simulink model "TorqueVect_HIL_CAN"  (R2022a)
settings: Solver=VariableStepAuto  StartTime=0.0  StopTime=300  RelTol=1e-3
PreLoadFcn:
  | run('Parameters\FSE_Parameters.m')
values from neighbouring files (symbols this model uses):
  Kd = 0;')    [open_carmaker_gui.m]
  Ki = 0    [open_carmaker_gui.m]
undefined symbols (not defined in the file or in its folder): BRegenEnabledButton, canChannel, CyalphaLookUp, efficiency, Fz_curve, Fz_scaling_long, gearR, izz, jw, kd, ki, Kp, kp, l_f, l_r, lambda, m, Mz_max, N, N_lat, N_long, P_max, pid_kd_lat, pid_kd_long, pid_ki_lat, pid_ki_long, pid_kp_lat, pid_kp_long, R_max, rw, steerR, T_i_max, TC_Decr_Gas, TC_Derivative, TC_Incr_Gas, TC_On, TC_Relay_Off, TC_Relay_On, tireCornerStiffness, Ts, TV_On, TV_Override, velocity_lookup, velocity_lookup_lat, y_ref, yrr_scaling
libraries: simulink x218, slpidlib x135, CarMaker4SL x73, TractionControlLibrary x13, canmsglib x11, canlib x10, TorqueVectoringLibrary x6, simulink_extras x4, PedalConversionLibrary x3, PowerControlLibrary x1
(part 2 of 26)

== system TorqueVect_HIL_CAN/CarMaker/IPG Vehicle/CarAndTrailer/Forces/Tires ==
  note: The TireXX_Out signals will only be used if FileIdent is "CarMaker-Tire-CM4SL" in the tire parameter file!
      | An example parameter file can be found in Data/Tire/DT_CM4SL_UserTire.
  Sync_In : Inport
  TireFL_In : Inport  Port=2
  TireFR_In : Inport  Port=3
  TireRL_In : Inport  Port=4
  TireRR_In : Inport  Port=5
  Bus Creator{1..4} (4 alike) : BusCreator  Inputs=11
  Demux{1..3,8} (4 alike) : Demux  Outputs=7
      settings: DisplayOption=none
  TireFL : Subsystem
  TireFR : Subsystem
  TireRL : Subsystem
  TireRR : Subsystem
  TireFL_Out : Outport
  TireFR_Out : Outport  Port=2
  TireRL_Out : Outport  Port=3
  TireRR_Out : Outport  Port=4
  tag scope: TireFL=global, TireFR=global, TireRL=global, TireRR=global
  wires:
  Sync_In/1 -> TireRR/1(Sync_In), TireRL/1(Sync_In), TireFR/1(Sync_In), TireFL/1(Sync_In)
  Bus Creator4/1 -> TireRR_Out/1
  Bus Creator2/1 -> TireRL_Out/1
  Bus Creator1/1 -> TireFR_Out/1
  Demux3/5 -> TireRR/6(Rim_turnv)  "Tire_In Rim_turnv"
  Demux3/4 -> TireRR/5(Rim_rotv)  "Tire_In Rim_rotv"
  Demux3/1 -> [TireRR], TireRR/2(Load)  "Tire_In Load"
  Demux3/7 -> TireRR/8(muRoad)  "Tire_In mu"
  Demux3/6 -> TireRR/7(InclinAngle)  "Tire_In Camber"
  Demux3/2 -> TireRR/3(vxtrans)  "Tire_In vxtrans"
  Demux3/3 -> TireRR/4(vytrans)  "Tire_In vytrans"
  TireRR/11(AlignTrq) -> Bus Creator4/11  "Tire_Out AlignTrq"
  TireRR/10(RollResist) -> Bus Creator4/10  "Tire_Out RollResist"
  TireRR/9(OverturnTrq) -> Bus Creator4/9  "Tire_Out OverturnTrq"
  TireRR/8(LoadFrc) -> Bus Creator4/8  "Tire_Out LoadFrc"
  TireRR/7(SideFrc) -> Bus Creator4/7  "Tire_Out SideFrc"
  TireRR/6(LongFrc) -> Bus Creator4/6  "Tire_Out LongFrc"
  TireRR/5(vBelt) -> Bus Creator4/5  "Tire_Out vBelt"
  TireRR/4(rBelt_eff) -> Bus Creator4/4  "Tire_Out rBelt_eff"
  TireRR/3(TurnSlp) -> Bus Creator4/3  "Tire_Out TurnSlp"
  TireRR/1(Slp) -> Bus Creator4/1  "Tire_Out Slp"
  TireRR/2(Alpha) -> Bus Creator4/2  "Tire_Out Alpha"
  Demux2/5 -> TireRL/6(Rim_turnv)  "Tire_In Rim_turnv"
  Demux2/4 -> TireRL/5(Rim_rotv)  "Tire_In Rim_rotv"
  Demux2/1 -> [TireRL], TireRL/2(Load)  "Tire_In Load"
  Demux2/7 -> TireRL/8(muRoad)  "Tire_In mu"
  Demux2/6 -> TireRL/7(InclinAngle)  "Tire_In Camber"
  Demux2/2 -> TireRL/3(vxtrans)  "Tire_In vxtrans"
  Demux2/3 -> TireRL/4(vytrans)  "Tire_In vytrans"
  TireRL/11(AlignTrq) -> Bus Creator2/11  "Tire_Out AlignTrq"
  TireRL/10(RollResist) -> Bus Creator2/10  "Tire_Out RollResist"
  TireRL/9(OverturnTrq) -> Bus Creator2/9  "Tire_Out OverturnTrq"
  TireRL/8(LoadFrc) -> Bus Creator2/8  "Tire_Out LoadFrc"
  TireRL/7(SideFrc) -> Bus Creator2/7  "Tire_Out SideFrc"
  TireRL/6(LongFrc) -> Bus Creator2/6  "Tire_Out LongFrc"
  TireRL/5(vBelt) -> Bus Creator2/5  "Tire_Out vBelt"
  TireRL/4(rBelt_eff) -> Bus Creator2/4  "Tire_Out rBelt_eff"
  TireRL/3(TurnSlp) -> Bus Creator2/3  "Tire_Out TurnSlp"
  TireRL/1(Slp) -> Bus Creator2/1  "Tire_Out Slp"
  TireRL/2(Alpha) -> Bus Creator2/2  "Tire_Out Alpha"
  Demux1/5 -> TireFR/6(Rim_turnv)  "Tire_In Rim_turnv"
  Demux1/4 -> TireFR/5(Rim_rotv)  "Tire_In Rim_rotv"
  Demux1/1 -> [TireFR], TireFR/2(Load)  "Tire_In Load"
  Demux1/7 -> TireFR/8(muRoad)  "Tire_In mu"
  Demux1/6 -> TireFR/7(InclinAngle)  "Tire_In Camber"
  Demux1/2 -> TireFR/3(vxtrans)  "Tire_In vxtrans"
  Demux1/3 -> TireFR/4(vytrans)  "Tire_In vytrans"
  TireFR/11(AlignTrq) -> Bus Creator1/11  "Tire_Out AlignTrq"
  TireFR/10(RollResist) -> Bus Creator1/10  "Tire_Out RollResist"
  TireFR/9(OverturnTrq) -> Bus Creator1/9  "Tire_Out OverturnTrq"
  TireFR/8(LoadFrc) -> Bus Creator1/8  "Tire_Out LoadFrc"
  TireFR/7(SideFrc) -> Bus Creator1/7  "Tire_Out SideFrc"
  TireFR/6(LongFrc) -> Bus Creator1/6  "Tire_Out LongFrc"
  TireFR/5(vBelt) -> Bus Creator1/5  "Tire_Out vBelt"
  TireFR/4(rBelt_eff) -> Bus Creator1/4  "Tire_Out rBelt_eff"
  TireFR/3(TurnSlp) -> Bus Creator1/3  "Tire_Out TurnSlp"
  TireFR/1(Slp) -> Bus Creator1/1  "Tire_Out Slp"
  TireFR/2(Alpha) -> Bus Creator1/2  "Tire_Out Alpha"
  Demux8/5 -> TireFL/6(Rim_turnv)  "Tire_In Rim_turnv"
  Demux8/4 -> TireFL/5(Rim_rotv)  "Tire_In Rim_rotv"
  TireFL_In/1 -> Demux8/1
  Demux8/1 -> [TireFL], TireFL/2(Load)  "Tire_In Load"
  Demux8/7 -> TireFL/8(muRoad)  "Tire_In mu"
  Demux8/6 -> TireFL/7(InclinAngle)  "Tire_In Camber"
  Demux8/2 -> TireFL/3(vxtrans)  "Tire_In vxtrans"
  Demux8/3 -> TireFL/4(vytrans)  "Tire_In vytrans"
  TireFL/11(AlignTrq) -> Bus Creator3/11  "Tire_Out AlignTrq"
  TireFL/10(RollResist) -> Bus Creator3/10  "Tire_Out RollResist"
  TireFL/9(OverturnTrq) -> Bus Creator3/9  "Tire_Out OverturnTrq"
  TireFL/8(LoadFrc) -> Bus Creator3/8  "Tire_Out LoadFrc"
  TireFL/7(SideFrc) -> Bus Creator3/7  "Tire_Out SideFrc"
  TireFL/6(LongFrc) -> Bus Creator3/6  "Tire_Out LongFrc"
  TireFL/5(vBelt) -> Bus Creator3/5  "Tire_Out vBelt"
  TireFL/4(rBelt_eff) -> Bus Creator3/4  "Tire_Out rBelt_eff"
  TireFL/3(TurnSlp) -> Bus Creator3/3  "Tire_Out TurnSlp"
  TireFL/1(Slp) -> Bus Creator3/1  "Tire_Out Slp"
  TireFL/2(Alpha) -> Bus Creator3/2  "Tire_Out Alpha"
  Bus Creator3/1 -> TireFL_Out/1
  TireFR_In/1 -> Demux1/1
  TireRL_In/1 -> Demux2/1
  TireRR_In/1 -> Demux3/1

== system TorqueVect_HIL_CAN/CarMaker/IPG Vehicle/CarAndTrailer/Forces/Vehicle Forces ==
  Sync_In : Inport
  Bus Creator1 : BusCreator  Inputs=12
  Bus Creator8 : BusCreator  Inputs=16
  BusCreator1 : BusCreator  Inputs=4
  BusCreator2 : BusCreator  Inputs=9
  Demux : Demux  Outputs=16
      settings: DisplayOption=none
  Demux1 : Demux  Outputs=12
      settings: DisplayOption=none
  Demux2 : Demux  Outputs=13
      settings: DisplayOption=none
  Forces : S-Function  FunctionName=CM_Sfun  Parameters='Forces'  SFunctionDeploymentMode=off  EnableBusSupport=off
  Terminator : Terminator
  Sync_Out : Outport
  Car.Virtual : Outport  Port=2
  Car.Aero : Outport  Port=3
  Car.Load : Outport  Port=4
  wires:
  BusCreator1/1 -> Terminator/1  "Aero IF (in)"
  Demux2/13 -> BusCreator2/9  "car Aero Trq_1 z"
  Demux2/12 -> BusCreator2/8  "car Aero Trq_1 y"
  Demux2/11 -> BusCreator2/7  "car Aero Trq_1 x"
  Demux2/10 -> BusCreator2/6  "car Aero Frc_1 z"
  Demux2/9 -> BusCreator2/5  "car Aero Frc_1 y"
  Demux2/8 -> BusCreator2/4  "car Aero Frc_1 x"
  Demux2/7 -> BusCreator2/3  "car Aero PoA_1 z"
  Demux2/6 -> BusCreator2/2  "car Aero PoA_1 y"
  Demux2/5 -> BusCreator2/1  "car Aero PoA_1 x"
  Demux2/4 -> BusCreator1/4  "car Aero tau_1"
  Demux2/3 -> BusCreator1/3  "car Aero ApproachVel_1 z"
  Demux2/2 -> BusCreator1/2  "car Aero ApproachVel_1 y"
  Demux2/1 -> BusCreator1/1  "car Aero ApproachVel_1 x"
  Demux/16 -> Bus Creator8/16  "Car Load_3 tz"
  Demux/15 -> Bus Creator8/15  "Car Load_3 ty"
  Demux/14 -> Bus Creator8/14  "Car Load_3 tx"
  Demux/13 -> Bus Creator8/13  "Car Load_3 mass"
  Demux1/12 -> Bus Creator1/12  "Car Virtual Trq_0 z"
  Demux1/11 -> Bus Creator1/11  "Car Virtual Trq_0 y"
  Demux1/10 -> Bus Creator1/10  "Car Virtual Trq_0 x"
  Demux1/9 -> Bus Creator1/9  "Car Virtual Trq_1 z"
  Demux1/8 -> Bus Creator1/8  "Car Virtual Trq_1 y"
  Demux1/7 -> Bus Creator1/7  "Car Virtual Trq_1 x"
  Demux1/6 -> Bus Creator1/6  "Car Virtual Frc_0 z"
  Demux1/5 -> Bus Creator1/5  "Car Virtual Frc_0 y"
  Demux1/4 -> Bus Creator1/4  "Car Virtual Frc_0 x"
  Sync_In/1 -> Forces/1
  Forces/1 -> Sync_Out/1
  BusCreator2/1 -> Car.Aero/1
  Demux1/1 -> Bus Creator1/1  "Car Virtual Frc_1 x"
  Demux1/2 -> Bus Creator1/2  "Car Virtual Frc_1 y"
  Demux1/3 -> Bus Creator1/3  "Car Virtual Frc_1 z"
  Forces/3 -> Demux2/1
  Forces/2 -> Demux1/1
  Bus Creator1/1 -> Car.Virtual/1
  Bus Creator8/1 -> Car.Load/1
  Demux/1 -> Bus Creator8/1  "Car Load_0 mass"
  Demux/2 -> Bus Creator8/2  "Car Load_0 tx"
  Demux/3 -> Bus Creator8/3  "Car Load_0 ty"
  Demux/4 -> Bus Creator8/4  "Car Load_0 tz"
  Demux/5 -> Bus Creator8/5  "Car Load_1 mass"
  Demux/6 -> Bus Creator8/6  "Car Load_1 tx"
  Demux/7 -> Bus Creator8/7  "Car Load_1 ty"
  Demux/8 -> Bus Creator8/8  "Car Load_1 tz"
  Demux/9 -> Bus Creator8/9  "Car Load_2 mass"
  Demux/10 -> Bus Creator8/10  "Car Load_2 tx"
  Demux/11 -> Bus Creator8/11  "Car Load_2 ty"
  Demux/12 -> Bus Creator8/12  "Car Load_2 tz"
  Forces/4 -> Demux/1

== system TorqueVect_HIL_CAN/CarMaker/IPG Vehicle/CarAndTrailer/Trailer/CreateBus Car.Hitch.FrcTrq ==
  In1 : Inport
  Bus Creator7 : BusCreator  Inputs=6
  Demux7 : Demux  Outputs=6
      settings: DisplayOption=none
  Out1 : Outport
  wires:
  In1/1 -> Demux7/1
  Bus Creator7/1 -> Out1/1
  Demux7/6 -> Bus Creator7/6  "Car Hitch Trq2Car z"
  Demux7/5 -> Bus Creator7/5  "Car Hitch Trq2Car y"
  Demux7/4 -> Bus Creator7/4  "Car Hitch Trq2Car x"
  Demux7/3 -> Bus Creator7/3  "Car Hitch Frc2Car z"
  Demux7/2 -> Bus Creator7/2  "Car Hitch Frc2Car y"
  Demux7/1 -> Bus Creator7/1  "Car Hitch Frc2Car x"

== system TorqueVect_HIL_CAN/CarMaker/IPG Vehicle/CarAndTrailer/Trailer/CreateBus Vhcl.Motion ==
  In1 : Inport
  BusCreator : BusCreator  Inputs=15
  Demux : Demux  Outputs=15
      settings: DisplayOption=none
  Out1 : Outport
  tag scope: yawVelCar=global
  wires:
  Demux/15 -> BusCreator/15  "Vhcl YawAcc"
  Demux/14 -> [yawVelCar], BusCreator/14  "Vhcl YawVel"
  Demux/13 -> BusCreator/13  "Vhcl Yaw"
  Demux/12 -> BusCreator/12  "Vhcl PitchAcc"
  Demux/11 -> BusCreator/11  "Vhcl PitchVel"
  Demux/10 -> BusCreator/10  "Vhcl Pitch"
  Demux/9 -> BusCreator/9  "Vhcl RollAcc"
  Demux/8 -> BusCreator/8  "Vhcl RollVel"
  Demux/7 -> BusCreator/7  "Vhcl Roll"
  Demux/6 -> BusCreator/6  "Vhcl Hitch_Pos z"
  Demux/5 -> BusCreator/5  "Vhcl Hitch_Pos y"
  Demux/4 -> BusCreator/4  "Vhcl Hitch_Pos x"
  Demux/3 -> BusCreator/3  "Vhcl sRoad"
  Demux/2 -> BusCreator/2  "Vhcl Distance"
  Demux/1 -> BusCreator/1  "Vhcl v"
  In1/1 -> Demux/1
  BusCreator/1 -> Out1/1

== system TorqueVect_HIL_CAN/CarMaker/IPG Vehicle/CarAndTrailer/Trailer/CreateBus Vhcl.PoI ==
  In1 : Inport
  Bus Creator3 : BusCreator  Inputs=18
  Demux3 : Demux  Outputs=18
      settings: DisplayOption=none
  Out1 : Outport
  tag scope: vehAccelx=global, vehAccely=global
  wires:
  Demux3/18 -> Bus Creator3/18  "Vhcl PoI_GCS Elev"
  Demux3/17 -> Bus Creator3/17  "Vhcl PoI_GCS Lat"
  Demux3/16 -> Bus Creator3/16  "Vhcl PoI_GCS Long"
  Demux3/15 -> Bus Creator3/15  "Vhcl PoI_Acc_1 z"
  Demux3/14 -> [vehAccely], Bus Creator3/14  "Vhcl PoI_Acc_1 y"
  Demux3/13 -> [vehAccelx], Bus Creator3/13  "Vhcl PoI_Acc_1 x"
  Demux3/12 -> Bus Creator3/12  "Vhcl PoI_Vel_1 z"
  Demux3/11 -> Bus Creator3/11  "Vhcl PoI_Vel_1 y"
  Demux3/10 -> Bus Creator3/10  "Vhcl PoI_Vel_1 x"
  Demux3/9 -> Bus Creator3/9  "Vhcl PoI_Acc z"
  Demux3/8 -> Bus Creator3/8  "Vhcl PoI_Acc y"
  Demux3/7 -> Bus Creator3/7  "Vhcl PoI_Acc x"
  Demux3/6 -> Bus Creator3/6  "Vhcl PoI_Vel z"
  Demux3/5 -> Bus Creator3/5  "Vhcl PoI_Vel y"
  Demux3/4 -> Bus Creator3/4  "Vhcl PoI_Vel x"
  Demux3/3 -> Bus Creator3/3  "Vhcl PoI_Pos z"
  Demux3/2 -> Bus Creator3/2  "Vhcl PoI_Pos y"
  In1/1 -> Demux3/1
  Bus Creator3/1 -> Out1/1
  Demux3/1 -> Bus Creator3/1  "Vhcl PoI_Pos x"

== system TorqueVect_HIL_CAN/CarMaker/IPG Vehicle/CarAndTrailer/Trailer/CreateBus Vhcl.Steering ==
  In1 : Inport
  Bus Creator3 : BusCreator  Inputs=4
  Demux : Demux
      settings: DisplayOption=none
  Out1 : Outport
  wires:
  Bus Creator3/1 -> Out1/1
  Demux/1 -> Bus Creator3/1  "Vhcl Steering Ang"
  Demux/3 -> Bus Creator3/3  "Vhcl Steering AngAcc"
  Demux/2 -> Bus Creator3/2  "Vhcl Steering AngVel"
  Demux/4 -> Bus Creator3/4  "Vhcl Steering Trq"
  In1/1 -> Demux/1

== system TorqueVect_HIL_CAN/CarMaker/IPG Vehicle/CarAndTrailer/Trailer/CreateBus Vhcl.Wheel.FL ==
  In1 : Inport
  Bus Creator3 : BusCreator  Inputs=14
  Demux3 : Demux  Outputs=14
      settings: DisplayOption=none
  Out1 : Outport
  wires:
  Demux3/14 -> Bus Creator3/14  "Vhcl Wheel FL Trq_WhlBearing"
  Demux3/13 -> Bus Creator3/13  "Vhcl Wheel FL Trq_T2W"
  Demux3/12 -> Bus Creator3/12  "Vhcl Wheel FL SideSlip"
  Demux3/11 -> Bus Creator3/11  "Vhcl Wheel FL LongSlip"
  Demux3/10 -> Bus Creator3/10  "Vhcl Wheel FL vBelt"
  Demux3/9 -> Bus Creator3/9  "Vhcl Wheel FL Fz"
  Demux3/8 -> Bus Creator3/8  "Vhcl Wheel FL Fy"
  Demux3/7 -> Bus Creator3/7  "Vhcl Wheel FL Fx"
  Demux3/6 -> Bus Creator3/6  "Vhcl Wheel FL r_zxy z"
  Demux3/5 -> Bus Creator3/5  "Vhcl Wheel FL r_zxy y"
  Demux3/4 -> Bus Creator3/4  "Vhcl Wheel FL r_zxy x"
  Demux3/3 -> Bus Creator3/3  "Vhcl Wheel FL t z"
  Demux3/2 -> Bus Creator3/2  "Vhcl Wheel FL t y"
  In1/1 -> Demux3/1
  Bus Creator3/1 -> Out1/1
  Demux3/1 -> Bus Creator3/1  "Vhcl Wheel FL t x"

== system TorqueVect_HIL_CAN/CarMaker/IPG Vehicle/CarAndTrailer/Trailer/CreateBus Vhcl.Wheel.FR ==
  In1 : Inport
  Bus Creator3 : BusCreator  Inputs=14
  Demux3 : Demux  Outputs=14
      settings: DisplayOption=none
  Out1 : Outport
  wires:
  Demux3/14 -> Bus Creator3/14  "Vhcl Wheel FR Trq_WhlBearing"
  Demux3/13 -> Bus Creator3/13  "Vhcl Wheel FR Trq_T2W"
  Demux3/12 -> Bus Creator3/12  "Vhcl Wheel FR SideSlip"
  Demux3/11 -> Bus Creator3/11  "Vhcl Wheel FR LongSlip"
  Demux3/10 -> Bus Creator3/10  "Vhcl Wheel FR vBelt"
  Demux3/9 -> Bus Creator3/9  "Vhcl Wheel FR Fz"
  Demux3/8 -> Bus Creator3/8  "Vhcl Wheel FR Fy"
  Demux3/7 -> Bus Creator3/7  "Vhcl Wheel FR Fx"
  Demux3/6 -> Bus Creator3/6  "Vhcl Wheel FR r_zxy z"
  Demux3/5 -> Bus Creator3/5  "Vhcl Wheel FR r_zxy y"
  Demux3/4 -> Bus Creator3/4  "Vhcl Wheel FR r_zxy x"
  Demux3/3 -> Bus Creator3/3  "Vhcl Wheel FR t z"
  Demux3/2 -> Bus Creator3/2  "Vhcl Wheel FR t y"
  In1/1 -> Demux3/1
  Bus Creator3/1 -> Out1/1
  Demux3/1 -> Bus Creator3/1  "Vhcl Wheel FR t x"

== system TorqueVect_HIL_CAN/CarMaker/IPG Vehicle/CarAndTrailer/Trailer/CreateBus Vhcl.Wheel.RL ==
  In1 : Inport
  Bus Creator3 : BusCreator  Inputs=14
  Demux3 : Demux  Outputs=14
      settings: DisplayOption=none
  Out1 : Outport
  wires:
  Demux3/14 -> Bus Creator3/14  "Vhcl Wheel RL Trq_WhlBearing"
  Demux3/13 -> Bus Creator3/13  "Vhcl Wheel RL Trq_T2W"
  Demux3/12 -> Bus Creator3/12  "Vhcl Wheel RL SideSlip"
  Demux3/11 -> Bus Creator3/11  "Vhcl Wheel RL LongSlip"
  Demux3/10 -> Bus Creator3/10  "Vhcl Wheel RL vBelt"
  Demux3/9 -> Bus Creator3/9  "Vhcl Wheel RL Fz"
  Demux3/8 -> Bus Creator3/8  "Vhcl Wheel RL Fy"
  Demux3/7 -> Bus Creator3/7  "Vhcl Wheel RL Fx"
  Demux3/6 -> Bus Creator3/6  "Vhcl Wheel RL r_zxy z"
  Demux3/5 -> Bus Creator3/5  "Vhcl Wheel RL r_zxy y"
  Demux3/4 -> Bus Creator3/4  "Vhcl Wheel RL r_zxy x"
  Demux3/3 -> Bus Creator3/3  "Vhcl Wheel RL t z"
  Demux3/2 -> Bus Creator3/2  "Vhcl Wheel RL t y"
  In1/1 -> Demux3/1
  Bus Creator3/1 -> Out1/1
  Demux3/1 -> Bus Creator3/1  "Vhcl Wheel RL t x"

== system TorqueVect_HIL_CAN/CarMaker/IPG Vehicle/CarAndTrailer/Trailer/CreateBus Vhcl.Wheel.RR ==
  In1 : Inport
  Bus Creator3 : BusCreator  Inputs=14
  Demux3 : Demux  Outputs=14
      settings: DisplayOption=none
  Out1 : Outport
  wires:
  Demux3/14 -> Bus Creator3/14  "Vhcl Wheel RR Trq_WhlBearing"
  Demux3/13 -> Bus Creator3/13  "Vhcl Wheel RR Trq_T2W"
  Demux3/12 -> Bus Creator3/12  "Vhcl Wheel RR SideSlip"
  Demux3/11 -> Bus Creator3/11  "Vhcl Wheel RR LongSlip"
  Demux3/10 -> Bus Creator3/10  "Vhcl Wheel RR vBelt"
  Demux3/9 -> Bus Creator3/9  "Vhcl Wheel RR Fz"
  Demux3/8 -> Bus Creator3/8  "Vhcl Wheel RR Fy"
  Demux3/7 -> Bus Creator3/7  "Vhcl Wheel RR Fx"
  Demux3/6 -> Bus Creator3/6  "Vhcl Wheel RR r_zxy z"
  Demux3/5 -> Bus Creator3/5  "Vhcl Wheel RR r_zxy y"
  Demux3/4 -> Bus Creator3/4  "Vhcl Wheel RR r_zxy x"
  Demux3/3 -> Bus Creator3/3  "Vhcl Wheel RR t z"
  Demux3/2 -> Bus Creator3/2  "Vhcl Wheel RR t y"
  In1/1 -> Demux3/1
  Bus Creator3/1 -> Out1/1
  Demux3/1 -> Bus Creator3/1  "Vhcl Wheel RR t x"

== system TorqueVect_HIL_CAN/CarMaker/IPG Vehicle/PowerTrain/PTControl Example/CreateBus PTC ClutchOut ==
  In : Inport
  BusCreator : BusCreator  Inputs=3
  Demux : Demux  Outputs=3
      settings: DisplayOption=none
  Out : Outport  VectorParamsAs1DForOutWhenUnconnected=off
  wires:
  In/1 -> Demux/1
  BusCreator/1 -> Out/1
  Demux/1 -> BusCreator/1  "PTC ClutchOut Pos"
  Demux/2 -> BusCreator/2  "PTC ClutchOut rotv_out_trg"
  Demux/3 -> BusCreator/3  "PTC ClutchOut Trq_out_trg"

== system TorqueVect_HIL_CAN/CarMaker/IPG Vehicle/PowerTrain/PTControl Example/CreateBus PTC EngineOut ==
  In : Inport
  BusCreator : BusCreator  Inputs=5
  Demux : Demux  Outputs=5
      settings: DisplayOption=none
  Out : Outport  VectorParamsAs1DForOutWhenUnconnected=off
  wires:
  In/1 -> Demux/1
  BusCreator/1 -> Out/1
  Demux/1 -> BusCreator/1  "PTC EngineOut set_ISC"
  Demux/2 -> BusCreator/2  "PTC EngineOut FuelCutOff"
  Demux/3 -> BusCreator/3  "PTC EngineOut Load"
  Demux/4 -> BusCreator/4  "PTC EngineOut Trq_trg"
  Demux/5 -> BusCreator/5  "PTC EngineOut rotv_trg"

== system TorqueVect_HIL_CAN/CarMaker/IPG Vehicle/PowerTrain/PTControl Example/CreateBus PTC GearBoxM_Out0 ==
  In : Inport
  BusCreator : BusCreator  Inputs=12
  Demux : Demux  Outputs=12
      settings: DisplayOption=none
  Out : Outport  PortDimensions=12  VectorParamsAs1DForOutWhenUnconnected=off
  wires:
  In/1 -> Demux/1
  BusCreator/1 -> Out/1
  Demux/1 -> BusCreator/1  "PTC GearBoxM_Out0 GearNoTrg"
  Demux/2 -> BusCreator/2  "PTC GearBoxM_Out0 GearNoTrg_dis"
  Demux/3 -> BusCreator/3  "PTC GearBoxM_Out0 set_ParkBrake"
  Demux/4 -> BusCreator/4  "PTC GearBoxM_Out0 i_trg"
  Demux/5 -> BusCreator/5  "PTC GearBoxM_Out0 rotv_in_trg"
  Demux/6 -> BusCreator/6  "PTC GearBoxM_Out0 Trq_out_trg"
  Demux/7 -> BusCreator/7  "PTC GearBoxM_Out0 Clutch Pos"
  Demux/8 -> BusCreator/8  "PTC GearBoxM_Out0 Clutch rotv_out_trg"
  Demux/9 -> BusCreator/9  "PTC GearBoxM_Out0 Clutch Trq_out_trg"
  Demux/10 -> BusCreator/10  "PTC GearBoxM_Out0 Clutch_dis Pos"
  Demux/11 -> BusCreator/11  "PTC GearBoxM_Out0 Clutch_dis rotv_out_trg"
  Demux/12 -> BusCreator/12  "PTC GearBoxM_Out0 Clutch_dis Trq_out_trg"

== system TorqueVect_HIL_CAN/CarMaker/IPG Vehicle/PowerTrain/PTControl Example/CreateBus PTC GearBoxM_Out1 ==
  In : Inport
  BusCreator : BusCreator  Inputs=12
  Demux : Demux  Outputs=12
      settings: DisplayOption=none
  Out : Outport  PortDimensions=12  VectorParamsAs1DForOutWhenUnconnected=off
  wires:
  In/1 -> Demux/1
  BusCreator/1 -> Out/1
  Demux/1 -> BusCreator/1  "PTC GearBoxM_Out1 GearNoTrg"
  Demux/2 -> BusCreator/2  "PTC GearBoxM_Out1 GearNoTrg_dis"
  Demux/3 -> BusCreator/3  "PTC GearBoxM_Out1 set_ParkBrake"
  Demux/4 -> BusCreator/4  "PTC GearBoxM_Out1 i_trg"
  Demux/5 -> BusCreator/5  "PTC GearBoxM_Out1 rotv_in_trg"
  Demux/6 -> BusCreator/6  "PTC GearBoxM_Out1 Trq_out_trg"
  Demux/7 -> BusCreator/7  "PTC GearBoxM_Out1 Clutch Pos"
  Demux/8 -> BusCreator/8  "PTC GearBoxM_Out1 Clutch rotv_out_trg"
  Demux/9 -> BusCreator/9  "PTC GearBoxM_Out1 Clutch Trq_out_trg"
  Demux/10 -> BusCreator/10  "PTC GearBoxM_Out1 Clutch_dis Pos"
  Demux/11 -> BusCreator/11  "PTC GearBoxM_Out1 Clutch_dis rotv_out_trg"
  Demux/12 -> BusCreator/12  "PTC GearBoxM_Out1 Clutch_dis Trq_out_trg"

== system TorqueVect_HIL_CAN/CarMaker/IPG Vehicle/PowerTrain/PTControl Example/CreateBus PTC GearBoxM_Out2 ==
  In : Inport
  BusCreator : BusCreator  Inputs=12
  Demux : Demux  Outputs=12
      settings: DisplayOption=none
  Out : Outport  PortDimensions=12  VectorParamsAs1DForOutWhenUnconnected=off
  wires:
  In/1 -> Demux/1
  BusCreator/1 -> Out/1
  Demux/1 -> BusCreator/1  "PTC GearBoxM_Out2 GearNoTrg"
  Demux/2 -> BusCreator/2  "PTC GearBoxM_Out2 GearNoTrg_dis"
  Demux/3 -> BusCreator/3  "PTC GearBoxM_Out2 set_ParkBrake"
  Demux/4 -> BusCreator/4  "PTC GearBoxM_Out2 i_trg"
  Demux/5 -> BusCreator/5  "PTC GearBoxM_Out2 rotv_in_trg"
  Demux/6 -> BusCreator/6  "PTC GearBoxM_Out2 Trq_out_trg"
  Demux/7 -> BusCreator/7  "PTC GearBoxM_Out2 Clutch Pos"
  Demux/8 -> BusCreator/8  "PTC GearBoxM_Out2 Clutch rotv_out_trg"
  Demux/9 -> BusCreator/9  "PTC GearBoxM_Out2 Clutch Trq_out_trg"
  Demux/10 -> BusCreator/10  "PTC GearBoxM_Out2 Clutch_dis Pos"
  Demux/11 -> BusCreator/11  "PTC GearBoxM_Out2 Clutch_dis rotv_out_trg"
  Demux/12 -> BusCreator/12  "PTC GearBoxM_Out2 Clutch_dis Trq_out_trg"

== system TorqueVect_HIL_CAN/CarMaker/IPG Vehicle/PowerTrain/PTControl Example/CreateBus PTC GearBoxM_Out3 ==
  In : Inport
  BusCreator : BusCreator  Inputs=12
  Demux : Demux  Outputs=12
      settings: DisplayOption=none
  Out : Outport  VectorParamsAs1DForOutWhenUnconnected=off
  wires:
  In/1 -> Demux/1
  BusCreator/1 -> Out/1
  Demux/1 -> BusCreator/1  "PTC GearBoxM_Out3 GearNoTrg"
  Demux/2 -> BusCreator/2  "PTC GearBoxM_Out3 GearNoTrg_dis"
  Demux/3 -> BusCreator/3  "PTC GearBoxM_Out3 set_ParkBrake"
  Demux/4 -> BusCreator/4  "PTC GearBoxM_Out3 i_trg"
  Demux/5 -> BusCreator/5  "PTC GearBoxM_Out3 rotv_in_trg"
  Demux/6 -> BusCreator/6  "PTC GearBoxM_Out3 Trq_out_trg"
  Demux/7 -> BusCreator/7  "PTC GearBoxM_Out3 Clutch Pos"
  Demux/8 -> BusCreator/8  "PTC GearBoxM_Out3 Clutch rotv_out_trg"
  Demux/9 -> BusCreator/9  "PTC GearBoxM_Out3 Clutch Trq_out_trg"
  Demux/10 -> BusCreator/10  "PTC GearBoxM_Out3 Clutch_dis Pos"
  Demux/11 -> BusCreator/11  "PTC GearBoxM_Out3 Clutch_dis rotv_out_trg"
  Demux/12 -> BusCreator/12  "PTC GearBoxM_Out3 Clutch_dis Trq_out_trg"

== system TorqueVect_HIL_CAN/CarMaker/IPG Vehicle/PowerTrain/PTControl Example/CreateBus PTC GearBoxOut ==
  In : Inport
  BusCreator : BusCreator  Inputs=12
  Demux : Demux  Outputs=12
      settings: DisplayOption=none
  Out : Outport  PortDimensions=12  VectorParamsAs1DForOutWhenUnconnected=off
  wires:
  In/1 -> Demux/1
  BusCreator/1 -> Out/1
  Demux/1 -> BusCreator/1  "PTC GearBoxOut GearNoTrg"
  Demux/2 -> BusCreator/2  "PTC GearBoxOut GearNoTrg_dis"
  Demux/3 -> BusCreator/3  "PTC GearBoxOut set_ParkBrake"
  Demux/4 -> BusCreator/4  "PTC GearBoxOut i_trg"
  Demux/5 -> BusCreator/5  "PTC GearBoxOut rotv_in_trg"
  Demux/6 -> BusCreator/6  "PTC GearBoxOut Trq_out_trg"
  Demux/7 -> BusCreator/7  "PTC GearBoxOut Clutch Pos"
  Demux/8 -> BusCreator/8  "PTC GearBoxOut Clutch rotv_out_trg"
  Demux/9 -> BusCreator/9  "PTC GearBoxOut Clutch Trq_out_trg"
  Demux/10 -> BusCreator/10  "PTC GearBoxOut Clutch_dis Pos"
  Demux/11 -> BusCreator/11  "PTC GearBoxOut Clutch_dis rotv_out_trg"
  Demux/12 -> BusCreator/12  "PTC GearBoxOut Clutch_dis Trq_out_trg"

== system TorqueVect_HIL_CAN/CarMaker/IPG Vehicle/PowerTrain/PTControl Example/CreateBus PTC ISGOut ==
  In : Inport
  BusCreator : BusCreator  Inputs=3
  Demux : Demux  Outputs=3
      settings: DisplayOption=none
  Out : Outport  VectorParamsAs1DForOutWhenUnconnected=off
  wires:
  In/1 -> Demux/1
  BusCreator/1 -> Out/1
  Demux/1 -> BusCreator/1  "PTC ISGOut Load"
  Demux/2 -> BusCreator/2  "PTC ISGOut Trq_trg"
  Demux/3 -> BusCreator/3  "PTC ISGOut rotv_trg"

== system TorqueVect_HIL_CAN/CarMaker/IPG Vehicle/PowerTrain/PTControl Example/CreateBus PTC MiscOut ==
  PTC MiscOut : Inport
  BusCreator : BusCreator  Inputs=4
  Demux : Demux
      settings: DisplayOption=none
  Out : Outport  VectorParamsAs1DForOutWhenUnconnected=off
  wires:
  PTC MiscOut/1 -> Demux/1
  BusCreator/1 -> Out/1
  Demux/1 -> BusCreator/1  "PTC_Out OperationState"
  Demux/2 -> BusCreator/2  "PTC_Out OperationError"
  Demux/3 -> BusCreator/3  "PTC_Out StrategyMode"
  Demux/4 -> BusCreator/4  "PTC_Out Ignition"

== system TorqueVect_HIL_CAN/CarMaker/IPG Vehicle/PowerTrain/PTControl Example/CreateBus PTC MotorOut0 ==
  MotorOut0 : Inport
  BusCreator : BusCreator  Inputs=3
  Demux : Demux  Outputs=3
      settings: DisplayOption=none
  Out : Outport  VectorParamsAs1DForOutWhenUnconnected=off
  wires:
  MotorOut0/1 -> Demux/1
  BusCreator/1 -> Out/1
  Demux/1 -> BusCreator/1  "PTC MotorOut0 Load"
  Demux/2 -> BusCreator/2  "PTC MotorOut0 Trq_trg"
  Demux/3 -> BusCreator/3  "PTC MotorOut0 rotv_trg"

== system TorqueVect_HIL_CAN/CarMaker/IPG Vehicle/PowerTrain/PTControl Example/CreateBus PTC MotorOut1 ==
  MotorOut1 : Inport
  BusCreator : BusCreator  Inputs=3
  Demux : Demux  Outputs=3
      settings: DisplayOption=none
  Out : Outport  VectorParamsAs1DForOutWhenUnconnected=off
  wires:
  MotorOut1/1 -> Demux/1
  BusCreator/1 -> Out/1
  Demux/1 -> BusCreator/1  "PTC MotorOut1 Load"
  Demux/2 -> BusCreator/2  "PTC MotorOut1 Trq_trg"
  Demux/3 -> BusCreator/3  "PTC MotorOut1 rotv_trg"

== system TorqueVect_HIL_CAN/CarMaker/IPG Vehicle/PowerTrain/PTControl Example/CreateBus PTC MotorOut2 ==
  MotorOut2 : Inport
  BusCreator : BusCreator  Inputs=3
  Demux : Demux  Outputs=3
      settings: DisplayOption=none
  Out : Outport  VectorParamsAs1DForOutWhenUnconnected=off
  wires:
  MotorOut2/1 -> Demux/1
  BusCreator/1 -> Out/1
  Demux/1 -> BusCreator/1  "PTC MotorOut2 Load"
  Demux/2 -> BusCreator/2  "PTC MotorOut2 Trq_trg"
  Demux/3 -> BusCreator/3  "PTC MotorOut2 rotv_trg"

== system TorqueVect_HIL_CAN/CarMaker/IPG Vehicle/PowerTrain/PTControl Example/CreateBus PTC MotorOut3 ==
  MotorOut3 : Inport
  BusCreator : BusCreator  Inputs=3
  Demux : Demux  Outputs=3
      settings: DisplayOption=none
  Out : Outport  VectorParamsAs1DForOutWhenUnconnected=off
  wires:
  MotorOut3/1 -> Demux/1
  BusCreator/1 -> Out/1
  Demux/1 -> BusCreator/1  "PTC MotorOut3 Load"
  Demux/2 -> BusCreator/2  "PTC MotorOut3 Trq_trg"
  Demux/3 -> BusCreator/3  "PTC MotorOut3 rotv_trg"

== system TorqueVect_HIL_CAN/CarMaker/IPG Vehicle/PowerTrain/PTControl Example/CreateBus PTC PwrSupplyOut ==
  In : Inport
  BusCreator : BusCreator  Inputs=1
  Demux : Demux  Outputs=1
      settings: DisplayOption=none
  Out : Outport  PortDimensions=1  VectorParamsAs1DForOutWhenUnconnected=off
  wires:
  In/1 -> Demux/1
  BusCreator/1 -> Out/1
  Demux/1 -> BusCreator/1  "PTC PwrSupplyOut Pwr_HV1toLV_trg"

== system TorqueVect_HIL_CAN/CarMaker/IPG Vehicle/PowerTrain/PTControl Example/CreateBus PTC WheelOut ==
  In : Inport
  BusCreator : BusCreator  Inputs=8
  Demux : Demux  Outputs=8
      settings: DisplayOption=none
  Out : Outport  PortDimensions=8  VectorParamsAs1DForOutWhenUnconnected=off
  wires:
  In/1 -> Demux/1
  BusCreator/1 -> Out/1
  Demux/1 -> BusCreator/1  "PTC WheelOut_FL Trq_BrakeReg"
  Demux/2 -> BusCreator/2  "PTC WheelOut_FL Trq_BrakeReg_max"
  Demux/3 -> BusCreator/3  "PTC WheelOut_FR Trq_BrakeReg"
  Demux/4 -> BusCreator/4  "PTC WheelOut_FR Trq_BrakeReg_max"
  Demux/5 -> BusCreator/5  "PTC WheelOut_RL Trq_BrakeReg"
  Demux/6 -> BusCreator/6  "PTC WheelOut_RL Trq_BrakeReg_max"
  Demux/7 -> BusCreator/7  "PTC WheelOut_RR Trq_BrakeReg"
  Demux/8 -> BusCreator/8  "PTC WheelOut_RR Trq_BrakeReg_max"

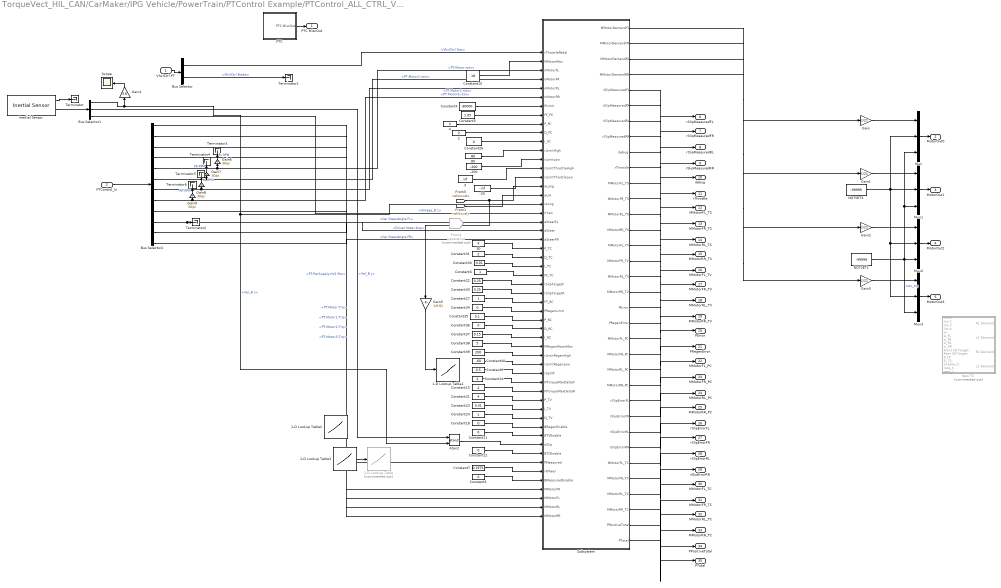
== system TorqueVect_HIL_CAN/CarMaker/IPG Vehicle/PowerTrain/PTControl Example/PTControl_ALL_CTRL_VC_MFE24 ==
  VhclCtrl.PT : Inport
  PTControl_In : Inport  Port=2
  -20 : Constant  Value=-inf
  -200 : Constant  Value=-200
  1-D Lookup Table : Lookup_n-D  Commented=on  NumberOfTableDimensions=1  BreakpointsForDimension1=[0 5 10 15 20]  Table=[0.3 0.3 0.3 0.3 0.3]  ExtrapMethod=Clip  InternalRulePriority=Speed  RndMeth=Simplest
  1-D Lookup Table1 : Lookup_n-D  NumberOfTableDimensions=1  BreakpointsForDimension1=[-1 -0.75 -0.5 -0.25 0 0.25 0.5 0.75 1]  Table=[0.75 0.65 0.58 0.525 0.5 0.475 0.42 0.3 0.2]  ExtrapMethod=Clip  InternalRulePriority=Speed  RndMeth=Simplest
  1-D Lookup Table2 : Lookup_n-D  NumberOfTableDimensions=1  BreakpointsForDimension1=[0 5 10]  Table=[0.1 0.4 0.4]  ExtrapMethod=Clip  InternalRulePriority=Speed  RndMeth=Simplest
  1-D Lookup Table3 : Lookup_n-D  NumberOfTableDimensions=1  BreakpointsForDimension1=[0 5 10 15 20]  Table=[0.1 0.3 0.42 0.475 0.5]  ExtrapMethod=Clip  InternalRulePriority=Speed  RndMeth=Simplest
  2 : Constant  Value=2
  3 : Constant  Value=inf
  30 : Constant  Value=4
  4 : Constant  Value=4
  80 : Constant  Value=80
  Atan2 : Trigonometry  Operator=atan2
  Bus Selector : BusSelector  OutputSignals=VhclCtrl Gas,VhclCtrl Brake
  Bus Selector1 : BusSelector  OutputSignals=Vel_B x,Vel_B y,Omega_B z
  Bus Selector2 : BusSelector  OutputSignals=PT:Motor.PT:Motor:Trq,PT:Motor.PT:Motor1:Trq,PT:Motor.PT:Motor2:Trq,PT:Motor.PT:Motor3:Trq,PT:Motor.PT:Motor:rotv,PT:Motor.PT:Motor1:rotv,PT:Motor.PT:Motor2:rotv,PT:Motor.PT:Motor3:rotv,PT:PwrSupply:HV1:Pwr,Steer.Driver:Steer:Ang,Steer.Car:SteerAngle:FL,Steer.Car:SteerAngle:FR
  Constant10 : Constant  Value=18
  Constant{3,11..12,18,26,34,36} (7 alike) : Constant  Value=0
  Constant14 : Constant  Value=2
  Constant15 : Constant  Value=2
  Constant21 : Constant  Value=4
  Constant22 : Constant  Value=0.25
  Constant23 : Constant  Value=0.01
  Constant24 : Constant
  Constant27 : Constant
  Constant30 : Constant  Value=0.01
  Constant31 : Constant  Value=2
  Constant33 : Constant  Value=0.25
  Constant35 : Constant  Value=0.1
  Constant37 : Constant  Value=0.15
  Constant38 : Constant  Value=5
  Constant39 : Constant  Value=200
  Constant4 : Constant  Value=80000
  Constant40 : Constant  Value=-60
  Constant5 : Constant  Value=1.05
  Constant6 : Constant
  Constant7 : Constant  Value=0.1975
  Constant9 : Constant  Value=0.5
  From4 : From  Commented=on  GotoTag=yawVelCar  TagVisibility=global
  Gain{,1..3} (4 alike) : Gain  Gain=1/21
  Gain4 : Gain  Gain=3.6
  Gain5 : Gain  Gain=1/9.81
  Gain{6..9} (4 alike) : Gain  Gain=30/pi
  Inertial Sensor : CarMaker4SL/Sensors/Inertial Sensor  xname=Param_B00  xstime=Continuous
      settings: SourceProductName=CarMaker4SL
  Mux{,1..3} (4 alike) : Mux  Inputs=3
  NOTSET1 : Constant  Value=-99999
  NOTSET3 : Constant  Value=-99999
  New TC : Subsystem  Commented=on
  PTC : Subsystem
  Scope : Scope
  Subsystem : Subsystem
  Terminator{,1..6} (7 alike) : Terminator
  PTC MiscOut : Outport  VectorParamsAs1DForOutWhenUnconnected=off
  MotorOut0 : Outport  Port=2  VectorParamsAs1DForOutWhenUnconnected=off
  MotorOut1 : Outport  Port=3  VectorParamsAs1DForOutWhenUnconnected=off
  MotorOut2 : Outport  Port=4  VectorParamsAs1DForOutWhenUnconnected=off
  MotorOut3 : Outport  Port=5  VectorParamsAs1DForOutWhenUnconnected=off
  rSlipMeasuredFL : Outport  Port=6
  rSlipMeasuredFR : Outport  Port=7
  rSlipMeasuredRL : Outport  Port=8
  rSlipMeasuredRR : Outport  Port=9
  debug : Outport  Port=10
  rThrottle : Outport  Port=11
  MMotorFL_TS : Outport  Port=12
  MMotorFR_TS : Outport  Port=13
  MMotorRL_TS : Outport  Port=14
  MMotorRR_TS : Outport  Port=15
  MMotorFL_TV : Outport  Port=16
  MMotorFR_TV : Outport  Port=17
  MMotorRL_TV : Outport  Port=18
  MMotorRR_TV : Outport  Port=19
  PError : Outport  Port=20
  PRegenError : Outport  Port=21
  MMotorFL_PC : Outport  Port=22
  MMotorFR_PC : Outport  Port=23
  MMotorRL_PC : Outport  Port=24
  MMotorRR_PC : Outport  Port=25
  rSlipErrorFL : Outport  Port=26
  rSlipErrorFR : Outport  Port=27
  rSlipErrorRL : Outport  Port=28
  rSlipErrorRR : Outport  Port=29
  MMotorFL_TC : Outport  Port=30
  MMotorFR_TC : Outport  Port=31
  MMotorRL_TC : Outport  Port=32
  MMotorRR_TC : Outport  Port=33
  PPositiveTotal : Outport  Port=34
  PTotal : Outport  Port=35
  wires:
  VhclCtrl.PT/1 -> Bus Selector/1
  PTC/1(PTC MiscOut) -> PTC MiscOut/1
  Inertial Sensor/2 -> Bus Selector1/1
  Bus Selector1/1 -> Subsystem/18(vLong), Atan2/2, Gain4/1  "<Vel_B x>"
  Inertial Sensor/1 -> Terminator/1
  Mux/1 -> MotorOut0/1
  Mux3/1 -> MotorOut3/1
  Mux2/1 -> MotorOut2/1
  Mux1/1 -> MotorOut1/1
  NOTSET3/1 -> Mux/2, Mux3/2, Mux2/2, Mux1/2
  NOTSET1/1 -> Mux/3, Mux1/3, Mux3/3, Mux2/3  "rotv_trg"
  Gain/1 -> Mux/1
  Gain1/1 -> Mux1/1
  Gain2/1 -> Mux2/1
  Gain3/1 -> Mux3/1
  Gain4/1 -> Scope/1
  3/1 -> Subsystem/14(rLimitThrottleHigh)
  Constant6/1 -> Subsystem/26(FF_TC)
  PTControl_In/1 -> Bus Selector2/1
  Subsystem/1(MMotorDemandFL) -> Gain/1
  Subsystem/2(MMotorDemandFR) -> Gain1/1
  Subsystem/3(MMotorDemandRL) -> Gain2/1
  Subsystem/4(MMotorDemandRR) -> Gain3/1
  Bus Selector2/1 -> Subsystem/50(MMotorFR)  "<PT:Motor:Trq>"
  Bus Selector2/2 -> Subsystem/51(MMotorFL)  "<PT:Motor1:Trq>"
  Bus Selector2/3 -> Subsystem/52(MMotorRL)  "<PT:Motor2:Trq>"
  Bus Selector2/4 -> Subsystem/53(MMotorRR)  "<PT:Motor3:Trq>"
  Bus Selector2/9 -> Subsystem/47(PMeasured)  "<PT:PwrSupply:HV1:Pwr>"
  Constant11/1 -> Subsystem/44(BTVEnable)
  Constant12/1 -> Subsystem/46(BTCEnable)
  Bus Selector2/5 -> Gain6/1, Subsystem/3(nMotorFL)  "<PT:Motor:rotv>"
  Bus Selector2/6 -> Gain7/1, Subsystem/4(nMotorFR)  "<PT:Motor1:rotv>"
  Bus Selector2/7 -> Gain8/1, Subsystem/5(nMotorRL)  "<PT:Motor2:rotv>"
  Bus Selector2/8 -> Gain9/1, Subsystem/6(nMotorRR)  "<PT:Motor3:rotv>"
  Constant14/1 -> Subsystem/38(NTorqueMaxDeltaF)
  Constant15/1 -> Subsystem/39(NTorqueMaxDeltaR)
  Bus Selector2/10 -> Subsystem/21(aSteer), Terminator2/1  "<Driver:Steer:Ang>"
  Constant18/1 -> Subsystem/43(BRegenEnable)
  Constant23/1 -> Subsystem/41(I_TV)
  Constant24/1 -> Subsystem/42(D_TV)
  Constant21/1 -> Subsystem/40(P_TV)
  Bus Selector/2 -> Terminator1/1  "<VhclCtrl Brake>"
  Bus Selector1/2 -> Atan2/1  "<Vel_B y>"
  Bus Selector/1 -> Subsystem/1(rThrottlePedal)  "<VhclCtrl Gas>"
  Bus Selector1/3 -> Subsystem/19(nYaw)  "<Omega_B z>"
  Bus Selector2/11 -> Subsystem/20(aSteerFL)  "<Car:SteerAngle:FL>"
  Bus Selector2/12 -> Subsystem/22(aSteerFR)  "<Car:SteerAngle:FR>"
  Subsystem/6(rSlipMeasuredFR) -> rSlipMeasuredFR/1
  Subsystem/25(rSlipErrorFL) -> rSlipErrorFL/1
  Subsystem/30(MMotorFR_TC) -> MMotorFR_TC/1
  Atan2/1 -> Subsystem/45(aSlip)
  Subsystem/14(MMotorRR_TS) -> MMotorRR_TS/1
  Subsystem/28(rSlipErrorRR) -> rSlipErrorRR/1
  Subsystem/31(MMotorRL_TC) -> MMotorRL_TC/1
  Subsystem/26(rSlipErrorFR) -> rSlipErrorFR/1
  Subsystem/19(PError) -> PError/1
  Subsystem/23(MMotorRL_PC) -> MMotorRL_PC/1
  Subsystem/16(MMotorFR_TV) -> MMotorFR_TV/1
  Subsystem/24(MMotorRR_PC) -> MMotorRR_PC/1
  Subsystem/29(MMotorFL_TC) -> MMotorFL_TC/1
  Subsystem/32(MMotorRR_TC) -> MMotorRR_TC/1
  Subsystem/8(rSlipMeasuredRR) -> rSlipMeasuredRR/1
  Subsystem/12(MMotorFR_TS) -> MMotorFR_TS/1
  Subsystem/34(PTotal) -> PTotal/1
  Subsystem/10(rThrottle) -> rThrottle/1
  Subsystem/21(MMotorFL_PC) -> MMotorFL_PC/1
  Subsystem/15(MMotorFL_TV) -> MMotorFL_TV/1
  Constant4/1 -> Subsystem/7(PLimit)
  Subsystem/7(rSlipMeasuredRL) -> rSlipMeasuredRL/1
  Subsystem/20(PRegenError) -> PRegenError/1
  Subsystem/22(MMotorFR_PC) -> MMotorFR_PC/1
  Subsystem/9(debug) -> debug/1
  Subsystem/5(rSlipMeasuredFL) -> rSlipMeasuredFL/1
  Subsystem/18(MMotorRR_TV) -> MMotorRR_TV/1
  Constant5/1 -> Subsystem/8(FF_PC)
  Constant10/1 -> Subsystem/2(MMotorMax)
  Subsystem/13(MMotorRL_TS) -> MMotorRL_TS/1
  Subsystem/11(MMotorFL_TS) -> MMotorFL_TS/1
  Subsystem/27(rSlipErrorRL) -> rSlipErrorRL/1
  Subsystem/17(MMotorRL_TV) -> MMotorRL_TV/1
  4/1 -> Subsystem/9(P_PC)
  Subsystem/33(PPositiveTotal) -> PPositiveTotal/1
  2/1 -> Subsystem/10(D_PC)
  Constant26/1 -> Subsystem/11(I_PC)
  80/1 -> Subsystem/12(rLimitHigh)
  -200/1 -> Subsystem/13(rLimitLow)
  30/1 -> Subsystem/23(P_TC)
  Constant31/1 -> Subsystem/24(D_TC)
  Constant30/1 -> Subsystem/25(I_TC)
  Constant22/1 -> Subsystem/27(rSlipTargetF)
  Constant33/1 -> Subsystem/28(rSlipTargetR)
  Constant27/1 -> Subsystem/29(FF_RC)
  Constant34/1 -> Subsystem/30(PRegenLimit)
  Constant35/1 -> Subsystem/31(P_RC)
  Constant36/1 -> Subsystem/32(D_RC)
  Constant37/1 -> Subsystem/33(I_RC)
  Constant38/1 -> Subsystem/34(MRegenMotorMax)
  Constant39/1 -> Subsystem/35(rLimitRegenHigh)
  Constant40/1 -> Subsystem/36(rLimitRegenLow)
  [vehAccelx] -> Gain5/1, Subsystem/16(aLong)
  Constant3/1 -> Subsystem/49(BMeasuredEnable)
  -20/1 -> Subsystem/15(rLimitThrottleLow)
  1-D Lookup Table3/1 -> 1-D Lookup Table/1
  Gain5/1 -> 1-D Lookup Table1/1
  Constant7/1 -> Subsystem/48(rWheel)
  Constant9/1 -> Subsystem/37(rSplitF)
  Gain6/1 -> Terminator3/1  "FL RPM"
  Gain8/1 -> Terminator5/1  "RL RPM"
  Gain7/1 -> Terminator4/1  "FR RPM"
  Gain9/1 -> Terminator6/1  "RR RPM"
  [vehAccely] -> Subsystem/17(aLat)

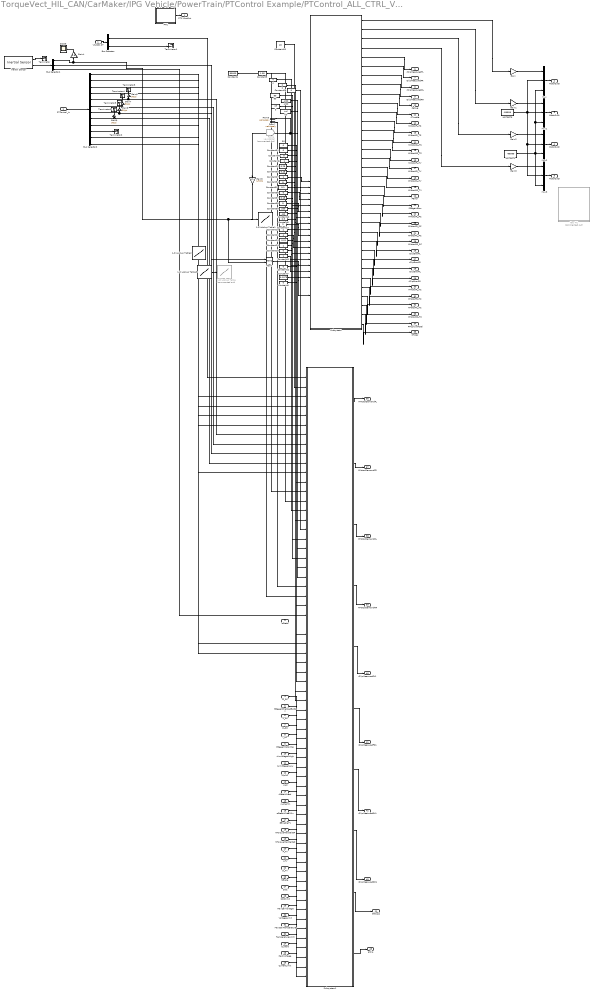
== system TorqueVect_HIL_CAN/CarMaker/IPG Vehicle/PowerTrain/PTControl Example/PTControl_ALL_CTRL_VC_REGEN ==
  VhclCtrl.PT : Inport
  PTControl_In : Inport  Port=2
  aSteer : Inport  Port=3
  FF_RC : Inport  Port=4
  BRegenEnabledButton : Inport  Port=5
  P_RC : Inport  Port=6
  D_RC : Inport  Port=7
  I_RC : Inport  Port=8
  MRegenMotorMax : Inport  Port=9
  rLimitRegenHigh : Inport  Port=10
  rLimitRegenLow : Inport  Port=11
  rSplitF : Inport  Port=12
  vLat : Inport  Port=13
  rSteerWheel : Inport  Port=14
  vLongMin : Inport  Port=15
  aSteerWheelMin : Inport  Port=16
  BEnableTV : Inport  Port=17
  NTorqueMaxDeltaF : Inport  Port=18
  NTorqueMaxDeltaR : Inport  Port=19
  P_TV : Inport  Port=20
  I_TV : Inport  Port=21
  D_TV : Inport  Port=22
  NBrake : Inport  Port=23
  Current : Inport  Port=24
  PackVoltage : Inport  Port=25
  CurrentLimit : Inport  Port=26
  SOC : Inport  Port=27
  SOClimit : Inport  Port=28
  MaxCellVoltage : Inport  Port=29
  VoltageLimit : Inport  Port=30
  MaxCellTemperature : Inport  Port=31
  TemperatureLimit : Inport  Port=32
  -20 : Constant  Value=-inf
  -200 : Constant  Value=-200
  1-D Lookup Table : Lookup_n-D  Commented=on  NumberOfTableDimensions=1  BreakpointsForDimension1=[0 5 10 15 20]  Table=[0.3 0.3 0.3 0.3 0.3]  ExtrapMethod=Clip  InternalRulePriority=Speed  RndMeth=Simplest
  1-D Lookup Table1 : Lookup_n-D  NumberOfTableDimensions=1  BreakpointsForDimension1=[-1 -0.75 -0.5 -0.25 0 0.25 0.5 0.75 1]  Table=[0.75 0.65 0.58 0.525 0.5 0.475 0.42 0.3 0.2]  ExtrapMethod=Clip  InternalRulePriority=Speed  RndMeth=Simplest
  1-D Lookup Table2 : Lookup_n-D  NumberOfTableDimensions=1  BreakpointsForDimension1=[0 5 10]  Table=[0.1 0.4 0.4]  ExtrapMethod=Clip  InternalRulePriority=Speed  RndMeth=Simplest
  1-D Lookup Table3 : Lookup_n-D  NumberOfTableDimensions=1  BreakpointsForDimension1=[0 5 10 15 20]  Table=[0.1 0.3 0.42 0.475 0.5]  ExtrapMethod=Clip  InternalRulePriority=Speed  RndMeth=Simplest
  2 : Constant  Value=2
  3 : Constant  Value=inf
  30 : Constant  Value=0
  4 : Constant  Value=4
  80 : Constant  Value=80
  Atan2 : Trigonometry  Operator=atan2
  Bus Selector : BusSelector  OutputSignals=VhclCtrl Gas,VhclCtrl Brake
  Bus Selector1 : BusSelector  OutputSignals=Vel_B x,Vel_B y,Omega_B z
  Bus Selector2 : BusSelector  OutputSignals=PT:Motor.PT:Motor:Trq,PT:Motor.PT:Motor1:Trq,PT:Motor.PT:Motor2:Trq,PT:Motor.PT:Motor3:Trq,PT:Motor.PT:Motor:rotv,PT:Motor.PT:Motor1:rotv,PT:Motor.PT:Motor2:rotv,PT:Motor.PT:Motor3:rotv,PT:PwrSupply:HV1:Pwr,Steer.Driver:Steer:Ang,Steer.Car:SteerAngle:FL,Steer.Car:SteerAngle:FR
  Constant10 : Constant  Value=18
  Constant{6,11,24,27} (4 alike) : Constant
  Constant{3,12,18,26,30..31,34,36} (8 alike) : Constant  Value=0
  Constant14 : Constant  Value=2
  Constant15 : Constant  Value=2
  Constant21 : Constant  Value=4
  Constant22 : Constant  Value=0.25
  Constant23 : Constant  Value=0.01
  Constant33 : Constant  Value=0.25
  Constant35 : Constant  Value=0.1
  Constant37 : Constant  Value=0.15
  Constant38 : Constant  Value=5
  Constant39 : Constant  Value=200
  Constant4 : Constant  Value=80000
  Constant40 : Constant  Value=-60
  Constant5 : Constant  Value=1.05
  Constant7 : Constant  Value=0.1975
  Constant9 : Constant  Value=0.5
  From4 : From  Commented=on  GotoTag=yawVelCar  TagVisibility=global
  Gain{,1..3} (4 alike) : Gain  Gain=1/21
  Gain4 : Gain  Gain=3.6
  Gain5 : Gain  Gain=1/9.81
  Gain{6..9} (4 alike) : Gain  Gain=30/pi
  Inertial Sensor : CarMaker4SL/Sensors/Inertial Sensor  xname=Param_B00  xstime=Continuous
      settings: SourceProductName=CarMaker4SL
  Mux{,1..3} (4 alike) : Mux  Inputs=3
  NOTSET1 : Constant  Value=-99999
  NOTSET3 : Constant  Value=-99999
  New TC : Subsystem  Commented=on
  PTC : Subsystem
  Scope : Scope
  Subsystem : Subsystem
  Subsystem1 : Subsystem
  Terminator{,1..6} (7 alike) : Terminator
  PTC MiscOut : Outport  VectorParamsAs1DForOutWhenUnconnected=off
  MotorOut0 : Outport  Port=2  VectorParamsAs1DForOutWhenUnconnected=off
  MotorOut1 : Outport  Port=3  VectorParamsAs1DForOutWhenUnconnected=off
  MotorOut2 : Outport  Port=4  VectorParamsAs1DForOutWhenUnconnected=off
  MotorOut3 : Outport  Port=5  VectorParamsAs1DForOutWhenUnconnected=off
  rSlipMeasuredFL : Outport  Port=6
  rSlipMeasuredFR : Outport  Port=7
  rSlipMeasuredRL : Outport  Port=8
  rSlipMeasuredRR : Outport  Port=9
  debug : Outport  Port=10
  rThrottle : Outport  Port=11
  MMotorFL_TS : Outport  Port=12
  MMotorFR_TS : Outport  Port=13
  MMotorRL_TS : Outport  Port=14
  MMotorRR_TS : Outport  Port=15
  MMotorFL_TV : Outport  Port=16
  MMotorFR_TV : Outport  Port=17
  MMotorRL_TV : Outport  Port=18
  MMotorRR_TV : Outport  Port=19
  PError : Outport  Port=20
  PRegenError : Outport  Port=21
  MMotorFL_PC : Outport  Port=22
  MMotorFR_PC : Outport  Port=23
  MMotorRL_PC : Outport  Port=24
  MMotorRR_PC : Outport  Port=25
  rSlipErrorFL : Outport  Port=26
  rSlipErrorFR : Outport  Port=27
  rSlipErrorRL : Outport  Port=28
  rSlipErrorRR : Outport  Port=29
  MMotorFL_TC : Outport  Port=30
  MMotorFR_TC : Outport  Port=31
  MMotorRL_TC : Outport  Port=32
  MMotorRR_TC : Outport  Port=33
  PPositiveTotal : Outport  Port=34
  PTotal : Outport  Port=35
  MMotorDemandFL : Outport  Port=36
  MMotorDemandFR : Outport  Port=37
  MMotorDemandRL : Outport  Port=38
  MMotorDemandRR : Outport  Port=39
  rSlipMeasuredFL1 : Outport  Port=40
  rSlipMeasuredFR1 : Outport  Port=41
  rSlipMeasuredRL1 : Outport  Port=42
  rSlipMeasuredRR1 : Outport  Port=43
  debug1 : Outport  Port=44
  aSlip : Outport  Port=45
  wires:
  VhclCtrl.PT/1 -> Bus Selector/1
  PTC/1(PTC MiscOut) -> PTC MiscOut/1
  Inertial Sensor/2 -> Bus Selector1/1
  Bus Selector1/1 -> Subsystem1/24(vLong), Atan2/2, Gain4/1  "<Vel_B x>"
  Inertial Sensor/1 -> Terminator/1
  Mux/1 -> MotorOut0/1
  Mux3/1 -> MotorOut3/1
  Mux2/1 -> MotorOut2/1
  Mux1/1 -> MotorOut1/1
  NOTSET3/1 -> Mux/2, Mux3/2, Mux2/2, Mux1/2
  NOTSET1/1 -> Mux/3, Mux1/3, Mux3/3, Mux2/3  "rotv_trg"
  Gain/1 -> Mux/1
  Gain1/1 -> Mux1/1
  Gain2/1 -> Mux2/1
  Gain3/1 -> Mux3/1
  Gain4/1 -> Scope/1
  3/1 -> Subsystem1/20(rLimitThrottleHigh)
  Constant6/1 -> Subsystem1/33(FF_TC)
  PTControl_In/1 -> Bus Selector2/1
  Subsystem/1(MMotorDemandFL) -> Gain/1
  Subsystem/2(MMotorDemandFR) -> Gain1/1
  Subsystem/3(MMotorDemandRL) -> Gain2/1
  Subsystem/4(MMotorDemandRR) -> Gain3/1
  Bus Selector2/1 -> Subsystem1/4(MMotorFR)  "<PT:Motor:Trq>"
  Bus Selector2/2 -> Subsystem1/3(MMotorFL)  "<PT:Motor1:Trq>"
  Bus Selector2/3 -> Subsystem1/5(MMotorRL)  "<PT:Motor2:Trq>"
  Bus Selector2/4 -> Subsystem1/6(MMotorRR)  "<PT:Motor3:Trq>"
  Bus Selector2/9 -> Subsystem1/11(PMeasured)  "<PT:PwrSupply:HV1:Pwr>"
  Constant11/1 -> Subsystem/43(BTVEnable)
  Constant12/1 -> Subsystem1/25(BEnableTC)
  Bus Selector2/5 -> Subsystem1/7(nMotorFL), Gain6/1  "<PT:Motor:rotv>"
  Bus Selector2/6 -> Subsystem1/8(nMotorFR), Gain7/1  "<PT:Motor1:rotv>"
  Bus Selector2/7 -> Subsystem1/9(nMotorRL), Gain8/1  "<PT:Motor2:rotv>"
  Bus Selector2/8 -> Subsystem1/10(nMotorRR), Gain9/1  "<PT:Motor3:rotv>"
  Constant14/1 -> Subsystem/37(NTorqueMaxDeltaF)
  Constant15/1 -> Subsystem/38(NTorqueMaxDeltaR)
  Bus Selector2/10 -> Terminator2/1  "<Driver:Steer:Ang>"
  Constant18/1 -> Subsystem/42(BRegenEnable)
  Constant23/1 -> Subsystem/40(I_TV)
  Constant24/1 -> Subsystem/41(D_TV)
  Constant21/1 -> Subsystem/39(P_TV)
  Bus Selector/2 -> Terminator1/1  "<VhclCtrl Brake>"
  Bus Selector1/2 -> Atan2/1  "<Vel_B y>"
  Bus Selector/1 -> Subsystem1/1(rThrottlePedal)  "<VhclCtrl Gas>"
  Bus Selector1/3 -> Subsystem1/26(nYaw)  "<Omega_B z>"
  Bus Selector2/11 -> Subsystem1/30(aSteerFL)  "<Car:SteerAngle:FL>"
  Bus Selector2/12 -> Subsystem1/29(aSteerFR)  "<Car:SteerAngle:FR>"
  Subsystem/6(rSlipMeasuredFR) -> rSlipMeasuredFR/1
  Subsystem/25(rSlipErrorFL) -> rSlipErrorFL/1
  Subsystem/30(MMotorFR_TC) -> MMotorFR_TC/1
  Atan2/1 -> Subsystem/44(aSlip)
  Subsystem/14(MMotorRR_TS) -> MMotorRR_TS/1
  Subsystem/28(rSlipErrorRR) -> rSlipErrorRR/1
  Subsystem/31(MMotorRL_TC) -> MMotorRL_TC/1
  Subsystem/26(rSlipErrorFR) -> rSlipErrorFR/1
  Subsystem/19(PError) -> PError/1
  Subsystem/23(MMotorRL_PC) -> MMotorRL_PC/1
  Subsystem/16(MMotorFR_TV) -> MMotorFR_TV/1
  Subsystem/24(MMotorRR_PC) -> MMotorRR_PC/1
  Subsystem/29(MMotorFL_TC) -> MMotorFL_TC/1
  Subsystem/32(MMotorRR_TC) -> MMotorRR_TC/1
  Subsystem/8(rSlipMeasuredRR) -> rSlipMeasuredRR/1
  Subsystem/12(MMotorFR_TS) -> MMotorFR_TS/1
  Subsystem/34(PTotal) -> PTotal/1
  Subsystem/10(rThrottle) -> rThrottle/1
  Subsystem/21(MMotorFL_PC) -> MMotorFL_PC/1
  Subsystem/15(MMotorFL_TV) -> MMotorFL_TV/1
  Constant4/1 -> Subsystem1/13(PLimit)
  Subsystem/7(rSlipMeasuredRL) -> rSlipMeasuredRL/1
  Subsystem/20(PRegenError) -> PRegenError/1
  Subsystem/22(MMotorFR_PC) -> MMotorFR_PC/1
  Subsystem/9(debug) -> debug/1
  Subsystem/5(rSlipMeasuredFL) -> rSlipMeasuredFL/1
  Subsystem/18(MMotorRR_TV) -> MMotorRR_TV/1
  Constant5/1 -> Subsystem1/14(FF_PC)
  Constant10/1 -> Subsystem1/2(MMotorMax)
  Subsystem/13(MMotorRL_TS) -> MMotorRL_TS/1
  Subsystem/11(MMotorFL_TS) -> MMotorFL_TS/1
  Subsystem/27(rSlipErrorRL) -> rSlipErrorRL/1
  Subsystem/17(MMotorRL_TV) -> MMotorRL_TV/1
  4/1 -> Subsystem1/15(P_PC)
  Subsystem/33(PPositiveTotal) -> PPositiveTotal/1
  2/1 -> Subsystem1/16(D_PC)
  Constant26/1 -> Subsystem1/17(I_PC)
  80/1 -> Subsystem1/18(rLimitHigh)
  -200/1 -> Subsystem1/19(rLimitLow)
  30/1 -> Subsystem1/28(P_TC)
  Constant31/1 -> Subsystem1/31(D_TC)
  Constant30/1 -> Subsystem1/32(I_TC)
  Constant22/1 -> Subsystem1/34(rSlipTargetF)
  Constant33/1 -> Subsystem1/35(rSlipTargetR)
  Constant27/1 -> Subsystem/28(FF_RC)
  Constant34/1 -> Subsystem/29(PRegenLimit)
  Constant35/1 -> Subsystem/30(P_RC)
  Constant36/1 -> Subsystem/31(D_RC)
  Constant37/1 -> Subsystem/32(I_RC)
  Constant38/1 -> Subsystem/33(MRegenMotorMax)
  Constant39/1 -> Subsystem/34(rLimitRegenHigh)
  Constant40/1 -> Subsystem/35(rLimitRegenLow)
  [vehAccelx] -> Subsystem1/22(aLong), Gain5/1
  Constant3/1 -> Subsystem1/12(BMeasuredEnable)
  -20/1 -> Subsystem1/21(rLimitThrottleLow)
  1-D Lookup Table3/1 -> 1-D Lookup Table/1
  Gain5/1 -> 1-D Lookup Table1/1
  Constant7/1 -> Subsystem/47(rWheel)
  Constant9/1 -> Subsystem/36(rSplitF)
  Gain6/1 -> Terminator3/1  "FL RPM"
  Gain8/1 -> Terminator5/1  "RL RPM"
  Gain7/1 -> Terminator4/1  "FR RPM"
  Gain9/1 -> Terminator6/1  "RR RPM"
  [vehAccely] -> Subsystem1/23(aLat)
  MaxCellVoltage/1 -> Subsystem1/58(MaxCellVoltage)
  vLongMin/1 -> Subsystem1/47(vLongMin)
  CurrentLimit/1 -> Subsystem1/64(CurrentLimit)
  NBrake/1 -> Subsystem1/55(NBrake)
  I_RC/1 -> Subsystem1/40(I_RC)
  rSteerWheel/1 -> Subsystem1/46(rSteerWheel)
  Subsystem1/4(MMotorDemandRR) -> MMotorDemandRR/1
  Subsystem1/5(rSlipMeasuredFL) -> rSlipMeasuredFL1/1
  P_RC/1 -> Subsystem1/38(P_RC)
  Current/1 -> Subsystem1/62(Current)
  BRegenEnabledButton/1 -> Subsystem1/37(BRegenEnabledButton)
  Subsystem1/3(MMotorDemandRL) -> MMotorDemandRL/1
  Subsystem1/1(MMotorDemandFL) -> MMotorDemandFL/1
  Subsystem1/7(rSlipMeasuredRL) -> rSlipMeasuredRL1/1
  Subsystem1/2(MMotorDemandFR) -> MMotorDemandFR/1
  rLimitRegenHigh/1 -> Subsystem1/42(rLimitRegenHigh)
  SOC/1 -> Subsystem1/56(SOC)
  VoltageLimit/1 -> Subsystem1/59(VoltageLimit)
  SOClimit/1 -> Subsystem1/57(SOClimit)
  MRegenMotorMax/1 -> Subsystem1/41(MRegenMotorMax)
  rLimitRegenLow/1 -> Subsystem1/43(rLimitRegenLow)
  Subsystem1/8(rSlipMeasuredRR) -> rSlipMeasuredRR1/1
  TemperatureLimit/1 -> Subsystem1/61(TemperatureLimit)
  FF_RC/1 -> Subsystem1/36(FF_RC)
  rSplitF/1 -> Subsystem1/44(rSplitF)
  aSteerWheelMin/1 -> Subsystem1/48(aSteerWheelMin)
  I_TV/1 -> Subsystem1/53(I_TV)
  NTorqueMaxDeltaF/1 -> Subsystem1/50(NTorqueMaxDeltaF)
  Subsystem1/9(debug) -> debug1/1
  Subsystem1/6(rSlipMeasuredFR) -> rSlipMeasuredFR1/1
  NTorqueMaxDeltaR/1 -> Subsystem1/51(NTorqueMaxDeltaR)
  MaxCellTemperature/1 -> Subsystem1/60(MaxCellTemperature)
  D_RC/1 -> Subsystem1/39(D_RC)
  D_TV/1 -> Subsystem1/54(D_TV)
  Subsystem1/10(aSlip) -> aSlip/1
  BEnableTV/1 -> Subsystem1/49(BTorqueVectoringEnable)
  PackVoltage/1 -> Subsystem1/63(PackVoltage)
  vLat/1 -> Subsystem1/45(vLat)
  P_TV/1 -> Subsystem1/52(P_TV)
